simulink model "zx_zitai"  (Simulink 6.2)
settings: Solver=ode3  StartTime=0.0  StopTime=10  FixedStep=0.005  RelTol=1e-3
values from neighbouring files (symbols this model uses):
  a22 = 0    [sim_3dof.m]
  a24 = (fy1(ma_cnt,alpha_cnt+1)-fy1(ma_cnt,alpha_cnt))/(alpha_vec(alpha_cnt+1)/57.3-alpha_vec(alpha_cnt)/57.3)/jz*Q*serf*L    [sim_3dof.m]    (also in trajnew.m = longchannel(:,10))
  a34 = (Ft+(l1(ma_cnt,alpha_cnt+1)-l1(ma_cnt,alpha_cnt))/(alpha_vec(alpha_cnt+1)/57.3-alpha_vec(alpha_cnt)/57.3)*Q*serf)/m/v    [sim_3dof.m]
  km = [-0.111852696169 -0.116507402631]    [zongxiang.mat]
  t1 = [27.3904972365 26.2990646017]    [zongxiang.mat]
  tm = [0.630563218333 0.601963031881]    [zongxiang.mat]
  ztam = [0.148183839315 0.147339242494]    [zongxiang.mat]
settings Model: LastModifiedBy=wangjsh
settings DebuggingCC: SolverPrmCheckMsg=warning

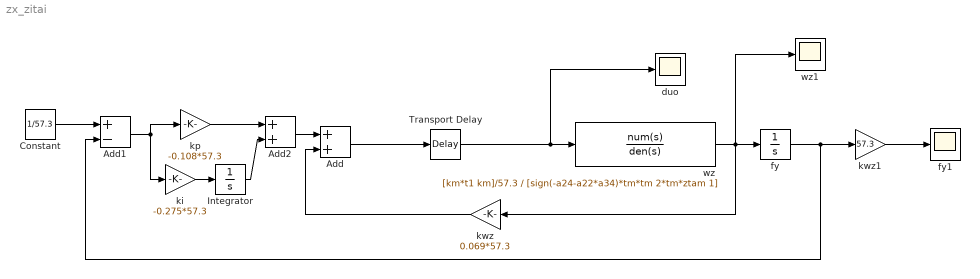
== system zx_zitai ==
  Add : Sum  OutScaling=2^-10
  Add1 : Sum  Inputs=+-  OutScaling=2^-10
  Add2 : Sum  OutScaling=2^-10
  Constant : Constant  Value=1/57.3
  Integrator : Integrator
  Transport Delay : TransportDelay  DelayTime=0
  duo : Scope
      settings: SaveName=ScopeData2
  fy : Integrator
  fy1 : Scope
  ki : Gain  Gain=-0.275*57.3
  kp : Gain  Gain=-0.108*57.3
  kwz : Gain  Orientation=left  Gain=0.069*57.3
  kwz1 : Gain  Gain=57.3
  wz : TransferFcn  Numerator=[km*t1 km]/57.3  Denominator=[sign(-a24-a22*a34)*tm*tm 2*tm*ztam 1]
  wz1 : Scope
  wires:
  wz/1 -> fy/1, wz1/1, kwz/1
  Add/1 -> Transport Delay/1
  kwz/1 -> Add/2
  fy/1 -> Add1/2, kwz1/1
  Constant/1 -> Add1/1
  Add2/1 -> Add/1
  Add1/1 -> kp/1, ki/1
  Integrator/1 -> Add2/2
  kp/1 -> Add2/1
  ki/1 -> Integrator/1
  Transport Delay/1 -> duo/1, wz/1
  kwz1/1 -> fy1/1
